simulink model "pvarray_mttp_sim_shading"  (R2021a)
settings: Solver=FixedStepAuto  StartTime=0.0  StopTime=0.4  FixedStep=1e-6  RelTol=1e-3  EnableMultiTasking=on
libraries: spsDiodeLib x4, spsSeriesRLCBranchLib x4, spsPVArrayLib x3, spsCurrentMeasurementLib x2, spsVoltageMeasurementLib x2, spsIGBTDiodeLib x1, spsPWMGeneratorDCDCLib x1, spspowerguiLib x1
settings Model: ExtModeTrigDuration=8  Creator=Federico  LastModifiedBy=Federico
settings SolverCC: AlgebraicLoopSolver=TrustRegion
settings OptimizationCC: DefaultUnderspecifiedDataType=single  EnhancedBackFolding=on  PassReuseOutputArgsAs=Individual arguments  MaxStackSize=1024  OptimizeBlockOrder=speed  DifferentSizesBufferReuse=on  OptimizationCustomize=off  DenormalBehavior=FlushToZero  EfficientTunableParamExpr=on
settings DebuggingCC: ParameterTunabilityLossMsg=error
settings HardwareCC: ProdBitPerChar=16  ProdBitPerInt=16  ProdBitPerPointer=32  ProdBitPerSizeT=32  ProdBitPerPtrDiffT=32  ProdLargestAtomicInteger=Integer  ProdLargestAtomicFloat=None  ProdWordSize=16  ProdLongLongMode=on  ProdHWDeviceType=Texas Instruments->C2000
settings ModelReferenceCC: ModelReferenceNumInstancesAllowed=Single
settings SFSimCC: MATLABDynamicMemAlloc=off
settings RTWCC: SystemTargetFile=ert.tlc  HardwareBoard=TI Delfino F28379D LaunchPad  TemplateMakefile=ert_default_tmf  Toolchain=Texas Instruments Code Composer Studio (C2000)  PortableWordSizes=on  CreateSILPILBlock=PIL  CodeExecutionProfiling=on  CodeProfilingInstrumentation=coarse
settings CodeAppCC: ForceParamTrailComments=on  IgnoreCustomStorageClasses=off  OperatorAnnotations=on  SimulinkDataObjDesc=on  SFDataObjDesc=on  InsertBlockDesc=on
settings ERTTargetCC: CodeReplacementLibrary=TI C28x  ExtModeTransport=4  ExtModeStaticAlloc=on  ExtModeMexFile=ext_xcp  ExtModeIntrfLevel=Level2 - Open

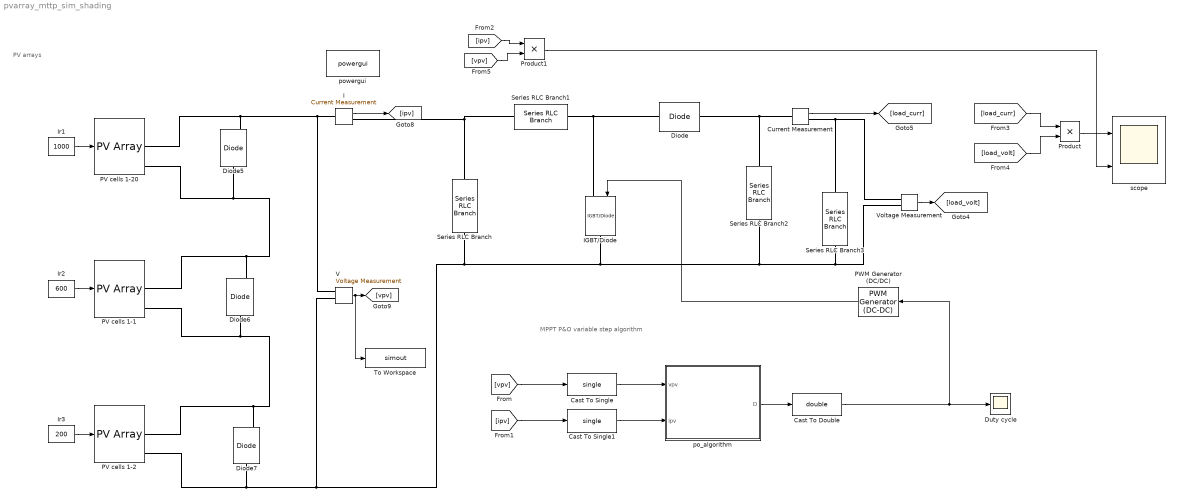
== system pvarray_mttp_sim_shading ==
  note: MPPT P&O variable step algorithm
  note: PV arrays
  Cast To Double : DataTypeConversion  OutDataTypeStr=double
  Cast To Single : DataTypeConversion  OutDataTypeStr=single
  Cast To Single1 : DataTypeConversion  OutDataTypeStr=single
  Current Measurement : spsCurrentMeasurementLib/Current Measurement  PhasorSimulation=off  OutputType=Complex  PSBequivalent=0
  Diode : spsDiodeLib/Diode  Ron=0.001  Lon=0  Vf=0.8  IC=0  UseSnubber=0  Rs=500  Cs=250e-9  Measurements=off
  Diode5 : spsDiodeLib/Diode  Ron=0.001  Lon=0  Vf=0.7  IC=0  UseSnubber=off  Rs=1e5*inf  Cs=inf  Measurements=on
  Diode6 : spsDiodeLib/Diode  Ron=0.001  Lon=0  Vf=0.7  IC=0  UseSnubber=off  Rs=1e5*inf  Cs=inf  Measurements=on
  Diode7 : spsDiodeLib/Diode  Ron=0.001  Lon=0  Vf=0.7  IC=0  UseSnubber=off  Rs=1e5*inf  Cs=inf  Measurements=on
  Duty cycle : Scope
  I : spsCurrentMeasurementLib/Current Measurement  PhasorSimulation=off  OutputType=Complex  PSBequivalent=0
  IGBT/Diode : spsIGBTDiodeLib/IGBT//Diode  Ron=1e-3  Rs=1e5  Cs=inf  Measurements=off
  Ir1 : Constant  Value=1000
  Ir2 : Constant  Value=600
  Ir3 : Constant  Value=200
  PV cells 1-1 : spsPVArrayLib/PV Array  Npar=64  Nser=2  PlotType=array @ 25 deg.C & specified irradiances  S_vec="[ 1000  300  600 ]"  Temp_C_vec="[ 45 25  ]"  ModuleName=User-defined  PlotWhenSelected=off  Pm=83.2824  Ncell=60/3  Voc=37.92*20/60  Isc=8.62  Vm=30.96*20/60  Im=8.07  beta_Voc_pc=-0.33969  alpha_Isc_pc=0.063701  beta_Voc=-0.042937  alpha_Isc=0.005491  IL=8.6307  I0=1.4176e-10  nI=0.99132  Rsh=82.1161  Rs=0.098625  RobustModel=on  RobustCellTemperature=25  BAL=on  Tc=1e-5  Tfilter=5e-5
      settings: AttributesFormatString=(%<RobustCellTemperature> deg.C)
  PV cells 1-2 : spsPVArrayLib/PV Array  Npar=64  Nser=1  PlotType=array @ 25 deg.C & specified irradiances  S_vec="[ 1000  300  600 ]"  Temp_C_vec="[ 45 25  ]"  ModuleName=User-defined  PlotWhenSelected=off  Pm=83.2824  Ncell=60/3  Voc=37.92*20/60  Isc=8.62  Vm=30.96*20/60  Im=8.07  beta_Voc_pc=-0.33969  alpha_Isc_pc=0.063701  beta_Voc=-0.042937  alpha_Isc=0.005491  IL=8.6307  I0=1.4176e-10  nI=0.99132  Rsh=82.1161  Rs=0.098625  RobustModel=on  RobustCellTemperature=25  BAL=on  Tc=1e-5  Tfilter=5e-5
      settings: AttributesFormatString=(%<RobustCellTemperature> deg.C)
  PV cells 1-20 : spsPVArrayLib/PV Array  Npar=64  Nser=2  PlotType=array @ 25 deg.C & specified irradiances  S_vec="[ 1000  300  600 ]"  Temp_C_vec="[ 45 25  ]"  ModuleName=SunPower SPR-315E-WHT-D  PlotWhenSelected=off  Pm=315.072  Ncell=96  Voc=64.6  Isc=6.14  Vm=54.7  Im=5.76  beta_Voc_pc=-0.2727  alpha_Isc_pc=0.061743  beta_Voc=-0.17616  alpha_Isc=0.003791  IL=6.1461  I0=6.5067e-12  nI=0.95071  Rsh=430.0666  Rs=0.43041  RobustModel=on  RobustCellTemperature=25  BAL=on  Tc=1e-5  Tfilter=5e-5
      settings: AttributesFormatString=(%<RobustCellTemperature> deg.C)
  PWM Generator (DC/DC) : spsPWMGeneratorDCDCLib/PWM Generator (DC-DC)  Fsw=5000  Ts=1e-6
  Product : Product
  Product1 : Product
  Series RLC Branch : spsSeriesRLCBranchLib/Series RLC Branch  LConnTagsString=__new0  RConnTagsString=__new0  BranchType=C  Resistance=1  Inductance=1e-3  SetiL0=off  InitialCurrent=0  Capacitance=100e-6  Setx0=off  InitialVoltage=0  Measurements=None
  Series RLC Branch1 : spsSeriesRLCBranchLib/Series RLC Branch  LConnTagsString=__new0  RConnTagsString=__new0  BranchType=L  Resistance=1  Inductance=5e-3  SetiL0=off  InitialCurrent=0  Capacitance=100e-6  Setx0=off  InitialVoltage=0  Measurements=None
  Series RLC Branch2 : spsSeriesRLCBranchLib/Series RLC Branch  LConnTagsString=__new0  RConnTagsString=__new0  BranchType=RC  Resistance=0.001  Inductance=3e-3  SetiL0=off  InitialCurrent=0  Capacitance=6000e-6  Setx0=off  InitialVoltage=0  Measurements=None
  Series RLC Branch3 : spsSeriesRLCBranchLib/Series RLC Branch  LConnTagsString=__new0  RConnTagsString=__new0  BranchType=R  Resistance=10  Inductance=3e-3  SetiL0=off  InitialCurrent=0  Capacitance=100e-6  Setx0=off  InitialVoltage=0  Measurements=None
  To Workspace : ToWorkspace  VariableName=simout  SaveFormat=Timeseries  SampleTime=-1
  V : spsVoltageMeasurementLib/Voltage Measurement  PhasorSimulation=off  OutputType=Complex  PSBequivalent=0
  Voltage Measurement : spsVoltageMeasurementLib/Voltage Measurement  PhasorSimulation=off  OutputType=Complex  PSBequivalent=0
  po_algorithm : MATLAB Function  TreatAsAtomicUnit=on
  powergui : spspowerguiLib/powergui  Priority=1  SimulationMode=Discrete  SampleTime=1e-6  frequency=60  Iterations=50  frequencyindice=0  Pbase=100e6  ErrMax=1e-4  UnitsV=kV  UnitsW=MW  buscounter=0  FunctionMessages=off  echomessages=off  EnableUseOfTLC=off  CurrentSourceSwitches=off  DisableSnubberDevices=off  DisableRonSwitches=off  DisableVfSwitches=off  DisplayEquations=off  AutomaticDiscreteSolvers=off  SolverType=Tustin/Backward Euler (TBE)  Interpol=off  ExternalGateDelay=off  methode=off  Ts=100  x0status=blocks  SPID=on  SwTol=0  HookPort=off  NonlinearTolerance=1e-4  nMaxIteration=100  ContinueOnMaxIteration=off  RestoreLinks=warning  ResistiveCurrentMeasurement=off  Frange=[0:2:500]  Ylog=off  Xlog=on  ShowGrid=off  save=off  variable=ZData  structure=0  ZoomFFT=off  StartTime=0.0  cycles=1  DisplayStyle=1  fundamental=60  FreqAxis=off  MaxFrequency=1000  frequencyindicesteady=1  RmsSteady=1  display=off
  scope : Scope  NumInputPorts=2
  wires:
  Current Measurement/1 -> [load_curr]
  Voltage Measurement/1 -> [load_volt]
  [load_curr] -> Product/1
  [load_volt] -> Product/2
  Product/1 -> scope/1
  Cast To Double/1 -> Duty cycle/1, PWM Generator (DC/DC)/1
  Cast To Single/1 -> po_algorithm/1(vpv)
  po_algorithm/1(D) -> Cast To Double/1
  Cast To Single1/1 -> po_algorithm/2(ipv)
  [vpv] -> Cast To Single/1
  [ipv] -> Cast To Single1/1
  Ir3/1 -> PV cells 1-2/1
  V/1 -> To Workspace/1, [vpv]
  I/1 -> [ipv]
  Ir1/1 -> PV cells 1-20/1
  Ir2/1 -> PV cells 1-1/1
  PWM Generator (DC/DC)/1 -> IGBT/Diode/1
  [ipv] -> Product1/1
  [vpv] -> Product1/2
  Product1/1 -> scope/2
  connections:
  Diode/LConn1 -- IGBT/Diode/LConn1 -- Series RLC Branch1/LConn1
  Current Measurement/LConn1 -- Series RLC Branch2/LConn1 -- Diode/RConn1
  Series RLC Branch3/RConn1 -- Current Measurement/RConn1 -- Voltage Measurement/LConn1
  Series RLC Branch1/RConn1 -- I/RConn1 -- Series RLC Branch/LConn1
  V/LConn2 -- PV cells 1-2/RConn2 -- Diode7/LConn1 -- Series RLC Branch2/RConn1 -- Series RLC Branch3/LConn1 -- Voltage Measurement/LConn2 -- IGBT/Diode/RConn1 -- Series RLC Branch/RConn1
  PV cells 1-20/RConn1 -- Diode5/RConn1 -- V/LConn1 -- I/LConn1
  Diode6/LConn1 -- PV cells 1-1/RConn2 -- PV cells 1-2/RConn1 -- Diode7/RConn1
  PV cells 1-1/RConn1 -- Diode6/RConn1 -- Diode5/LConn1 -- PV cells 1-20/RConn2

== matlab function pvarray_mttp_sim_shading/po_algorithm ==
  data: vpv input; D output; ipv input
function D = PO_algorithm(vpv, ipv)
    Dinit =single(0.4);
    Dmax = single(0.9);
    Dmin = single(0.1);
    
    persistent Vold Pold Dold
     
    if isempty(Vold)
        Vold = single(0);
        Pold = single(0);
        Dold = single(Dinit);
    end
    
    P = single(vpv*ipv);
    dV = vpv - Vold;
    dP = P - Pold; 
    N = 6e-6; %6e-6 funziona bene
    D_incr = single(N*abs(dP)); %VARIABLE
    %D_incr = 1e-5;
    
   
    if dP ~= 0
        if dP < 0
            if dV < 0
                D = Dold - D_incr;
            else
                D = Dold + D_incr;
            end
        else
            if dV < 0
                D = Dold + D_incr;
            else
                D = Dold - D_incr;
            end
        end
    else
        D = Dold;
    end
    
    if D >= Dmax || D <= Dmin
        D = Dold;
    end
    
    Dold = D;
    Vold = vpv;
    Pold = P;
           
end
